simulink model "Simulink_Blocks"  (R2025b)
settings: Solver=FixedStepAuto  StartTime=0.0  StopTime=inf  RelTol=1e-3
undefined symbols (not defined in the file): Hermitian, j, jsin, magnitude, Skew, Symmetric
libraries: simulink x38, matrix_library x7
settings Model: SimulationMode=external  Creator=kueh_js  LastModifiedBy=kueh_js
settings OptimizationCC: OptimizeBlockIOStorage=off  EnhancedBackFolding=on  PassReuseOutputArgsThreshold=0.0  ZeroExternalMemoryAtStartup=off  ZeroInternalMemoryAtStartup=off  OptimizeBlockOrder=speed  DifferentSizesBufferReuse=on
settings DebuggingCC: ParameterTunabilityLossMsg=error
settings HardwareCC: ProdBitPerLong=64.0  ProdHWDeviceType=Intel->x86-64 (Linux 64)
settings SFSimCC: MATLABDynamicMemAlloc=off  SimTargetLang=C++  SimDLTargetLibrary=mkl-dnn
settings RTWCC: GenCodeOnly=on  Toolchain=GNU gcc/g++ | gmake (64-bit Linux)  TargetLang=C++
settings CodeAppCC: ForceParamTrailComments=on  OperatorAnnotations=on  MATLABSourceComments=on
settings GRTTargetCC: TargetLangStandard=C++20 (ISO)  MatFileLogging=off  CodeInterfacePackaging=C++ class

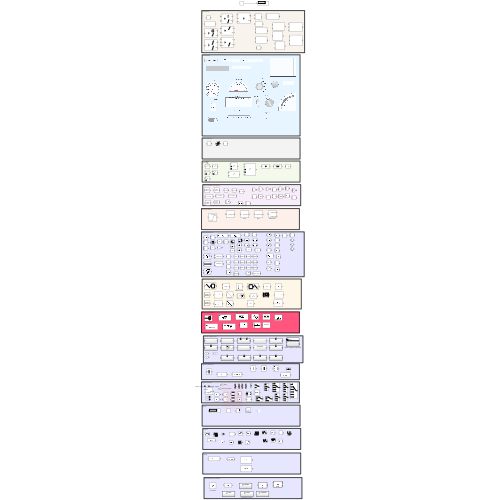
[thumbnail: Simulink's stored preview of the top-level diagram]
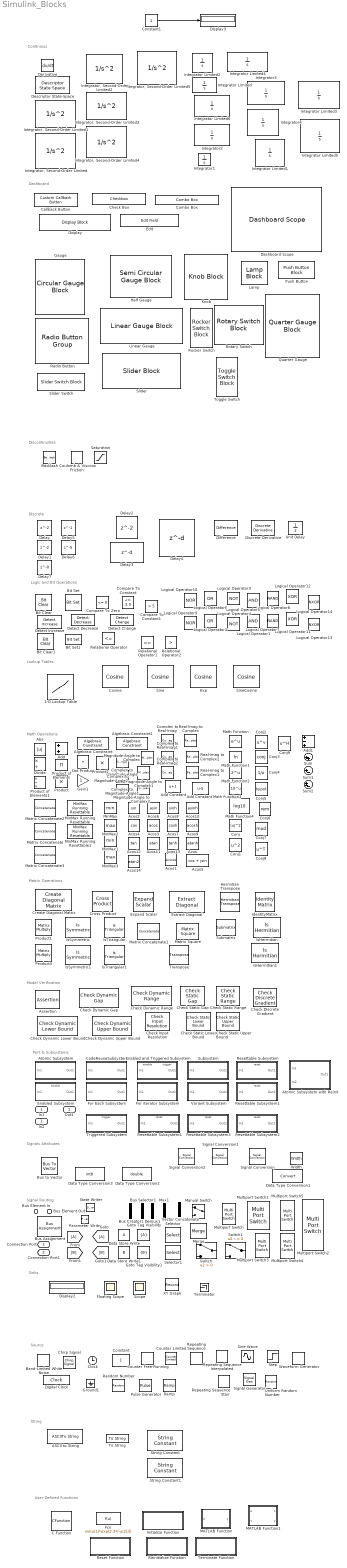
== system Simulink_Blocks ==
  note: Discontinuities
  note: Dashboard
  note: Continious
  note: Discrete
  note: Logic and Bit Operations
  note: Lookup Tables
  note: Math Operations
  note: Matrix Operations
  note: Model Verification
  note: Port & Subsystems
  note: Signals Attributes
  note: Signal Routing
  note: Sinks
  note: Source
  note: String
  note: User-Defined Functions
  In1 : Inport
  Bus Element In : Inport  Port=2  PortName=InBus  Element=signal1
  1-D Lookup Table : Lookup_n-D  NumberOfTableDimensions=1  BreakpointsForDimension1=[-5:5]  Table=tanh([-5:5])  InternalRulePriority=Speed  RndMeth=Simplest
  ASCII to String : ASCIIToString
  Abs : Abs  SaturateOnIntegerOverflow=off
  Acos : Trigonometry  Operator=atanh
  Acos1 : Trigonometry  Operator=sincos
  Acos10 : Trigonometry  Operator=asinh
  Acos11 : Trigonometry  Operator=atan
  Acos12 : Trigonometry  Operator=tan
  Acos13 : Trigonometry  Operator=tanh
  Acos14 : Trigonometry  Operator=atan2
  Acos2 : Trigonometry
  Acos3 : Trigonometry  Operator=acos
  Acos4 : Trigonometry  Operator=cos
  Acos5 : Trigonometry  Operator=cos + jsin
  Acos6 : Trigonometry  Operator=asin
  Acos7 : Trigonometry  Operator=cosh
  Acos8 : Trigonometry  Operator=sinh
  Acos9 : Trigonometry  Operator=acosh
  Add : Sum
  Add Constant : Bias  Bias=1  SaturateOnIntegerOverflow=off
  Add Constant1 : Bias  Bias=-5  SaturateOnIntegerOverflow=off
  Add1 : Sum  Inputs=+-+
  Algebraic Constraint : AlgebraicConstraint
  Algebraic Constraint1 : AlgebraicConstraint  Constraint=f(z) = z
  Assertion : Assertion
  Atomic Subsystem : Subsystem  TreatAsAtomicUnit=on
  Atomic Subsystem with Reinit : Subsystem  TreatAsAtomicUnit=on  ShowSubsystemReinitializePorts=on
  Backlash : Backlash
  Band-Limited White Noise : simulink/Sources/Band-Limited White Noise  Cov=[0.1]  Ts=0.1  seed=[23341]
  Bit Clear : simulink/Logic and Bit Operations/Bit Clear  iBit=0
  Bit Clear1 : simulink/Logic and Bit Operations/Bit Clear  iBit=3
  Bit Set : simulink/Logic and Bit Operations/Bit Set  iBit=0
  Bit Set1 : simulink/Logic and Bit Operations/Bit Set  iBit=2
  Bus Assignment : BusAssignment  AssignedSignals=signal1
  Bus Creator1 : BusCreator  Inputs=2
  Bus Selector1 : BusSelector  OutputSignals=signal1,signal2
  Bus to Vector : BusToVector
  C Function : CFunction
  Callback Button : CustomCallbackButton  Configuration="{\"components\":[{\"name\":\"BackgroundImageComponent\",\"settings\":{\"image\":{\"size\":[0,0],\"src\":\"default\",\"srcOrientation\":\"Right\"},\"position\":[0,0,1,1]}},{\"name\":\"ButtonStateComponent\",\"settings\":{\"buttonType\":\"momentary\",\"clickFcn\":\"\",\"onValue\":1,\"position\":[0,0,1,1],\"pressDelay\":\"500\",\"pressFcn\":\"\",\"repeatInterval\":\"0\",\"states\":[{\"horizontalAlignment\":\"center\",\"image\":{\"position\":[0,0,1,1],\"src\":\"default\",\"srcOrientation\":\"Right\"},\"label\":{\"color\":[0.01176470588,0.01176470588,0.01176470588,1],\"icon\":{\"size\":[0,0],\"src\":\"default\",\"srcOrientation\":\"Right\"},\"iconPlacement\":\"left\",\"text\":{\"content\":\"Callback Button\"}},\"labelOffset\":[0,0],\"verticalAlignment\":\"middle\"},{\"horizontalAlignment\":\"center\",\"image\":{\"position\":[0,0,1,1],\"src\":\"default\",\"srcOrientation\":\"Right\"},\"label\":{\"color\":[0.01176470588,0.01176470588,0.01176470588,1],\"icon\":{\"size\":[0,0],\"src\":\"default\",\"srcOrientation\":\"Right\"},\"iconPlacement\":\"left\",\"text\":{\"content\":\"Callback Button\"}},\"labelOffset\":[0,0],\"verticalAlignment\":\"middle\"},{\"horizontalAlignment\":\"center\",\"image\":{\"position\":[0,0,1,1],\"src\":\"default\",\"srcOrientation\":\"Right\"},\"label\":{\"color\":[0.01176470588,0.01176470588,0.01176470588,1],\"icon\":{\"size\":[0,0],\"src\":\"default\",\"srcOrientation\":\"Right\"},\"iconPlacement\":\"left\",\"text\":{\"content\":\"Callback Button\"}},\"labelOffset\":[0,0],\"verticalAlignment\":\"middle\"},{\"horizontalAlignment\":\"center\",\"image\":{\"position\":[0,0,1,1],\"src\":\"default\",\"srcOrientation\":\"Right\"},\"label\":{\"color\":[0.01176470588,0.01176470588,0.01176470588,1],\"icon\":{\"size\":[0,0],\"src\":\"default\",\"srcOrientation\":\"Right\"},\"iconPlacement\":\"left\",\"text\":{\"content\":\"Callback Button\"}},\"labelOffset\":[0,0],\"verticalAlignment\":\"middle\"}]}},{\"name\":\"ForegroundImageComponent\",\"settings\":{\"image\":{\"size\":[0,0],\"src\":\"default\",\"srcOrientation\":\"Right\"},\"isForeground\":1,\"position\":[0,0,1,1]}}],\"derived\":{\"blockParameters\":{\"AutoActivate\":true,\"ButtonText\":\"Callback Button\",\"ButtonType\":\"Momentary\",\"ClickFcn\":\"\",\"OnValue\":1,\"PressDelay\":\"500\",\"PressFcn\":\"\",\"RepeatInterval\":\"0\",\"fixedAspectRatio\":\"off\"}},\"settings\":{\"BindingType\":\"standalone\",\"autoActivate\":true,\"backgroundColor\":[244,244,244,1],\"backgroundOffset\":0.2,\"backgroundOpacity\":1,\"fixedAspectRatio\":\"off\",\"foregroundColor\":[0.01176470588,0.01176470588,0.01176470588,1],\"migratedFromLegacy\":true,\"useBackgroundColor\":true,\"variant\":\"callback\",\"version\":\"R2025a\"},\"type\":\"Button\"}"  CustomBackgroundColor="{\"color\":[0.9568627451,0.9568627451,0.9568627451],\"show\":true}"
  Check Discrete Gradient : simulink/Model Verification/Check Discrete Gradient  Description=| du / dt | < 1  gradient=1  enabled=on  stopWhenAssertionFail=on  export=off  icon=graphic
  Check Dynamic Gap : simulink/Model Verification/Check  Dynamic Gap  Description=u < min || max < u  enabled=on  stopWhenAssertionFail=on  export=off  icon=graphic
  Check Dynamic Range : simulink/Model Verification/Check  Dynamic Range  Description=min < u < max  enabled=on  stopWhenAssertionFail=on  export=off  icon=graphic
  Check Static Gap : simulink/Model Verification/Check  Static Gap  Description=u <= 0 || 100 <= u  max=100  max_included=on  min=0  min_included=on  enabled=on  stopWhenAssertionFail=on  export=off  icon=graphic
  Check Static Range : simulink/Model Verification/Check  Static Range  Description=0 <= u <= 100  max=100  max_included=on  min=0  min_included=on  enabled=on  stopWhenAssertionFail=on  export=off  icon=graphic
  Check Box : Checkbox  LabelPosition=Hide  ShowInitialText=on  Values=[0.0, 1.0]
  Check Dynamic Lower Bound : simulink/Model Verification/Check Dynamic  Lower Bound  Description=min < u  Enabled=on  stopWhenAssertionFail=on  export=off  icon=graphic
  Check Dynamic Upper Bound : simulink/Model Verification/Check Dynamic  Upper Bound  Description=u < max  enabled=on  stopWhenAssertionFail=on  export=off  icon=graphic
  Check Input Resolution : simulink/Model Verification/Check Input  Resolution  Description=-Inf < u < +Inf  resolution=1  enabled=on  stopWhenAssertionFail=on  export=off
  Check Static Lower Bound : simulink/Model Verification/Check Static  Lower Bound  Description=0 <= u  min=0  min_included=on  enabled=on  stopWhenAssertionFail=on  export=off  icon=graphic
  Check Static Upper Bound : simulink/Model Verification/Check Static  Upper Bound  Description=u <= 0  max=0  max_included=on  enabled=on  stopWhenAssertionFail=on  export=off  icon=graphic
  Chirp Signal : simulink/Sources/Chirp Signal  f1=0.1  T=100  f2=1
  Clock : Clock
  CodeReuseSubsystem : Subsystem  TreatAsAtomicUnit=on
      settings: RTWFcnNameOpts=Use subsystem name  RTWFileNameOpts=Use function name
  Combo Box : ComboBox  LabelPosition=Hide  SelectedLabel=Label2
  Compare To Constant : simulink/Logic and Bit Operations/Compare To Constant  relop=<=  const=3.0  OutDataTypeStr=boolean
  Compare To Constant1 : simulink/Logic and Bit Operations/Compare To Constant  relop=>  const=5  OutDataTypeStr=boolean
  Compare To Zero : simulink/Logic and Bit Operations/Compare To Zero  relop=<=  OutDataTypeStr=boolean
  Complex to Magnitude-Angle : ComplexToMagnitudeAngle
  Complex to Magnitude-Angle1 : ComplexToMagnitudeAngle  Output=Angle
  Complex to Magnitude-Angle2 : ComplexToMagnitudeAngle  Output=Magnitude
  Complex to Real-Imag : ComplexToRealImag
  Complex to Real-Imag1 : ComplexToRealImag  Output=Real
  Complex to Real-Imag2 : ComplexToRealImag  Output=Imag
  Conj : Math  Operator=magnitude^2
  Conj1 : Math  Operator=square
  Conj2 : Math  Operator=pow
  Conj3 : Math  Operator=conj
  Conj4 : Math  Operator=reciprocal
  Conj5 : Math  Operator=hypot
  Conj6 : Math  Operator=rem
  Conj7 : Math  Operator=mod
  Conj8 : Math  Operator=transpose
  Conj9 : Math  Operator=hermitian
  Constant : Constant
  Constant1 : Constant
  Cosine : simulink/Lookup Tables/Cosine  Formula=cos(2*pi*u)  NumDataPoints=(2^5)+1  OutputWordLength=16  InternalRulePriority=Speed
  Coulomb & Viscous Friction : simulink/Discontinuities/Coulomb & Viscous Friction  offset=[1 3 2 0]  gain=1
  Counter Free-Running : simulink/Sources/Counter Free-Running  NumBits=16  tsamp=-1
  Counter Limited : simulink/Sources/Counter Limited  uplimit=7  tsamp=-1
  Create Diagonal Matrix : matrix_library/Create Diagonal Matrix
      settings: LibrarySourceBlock=|
      | simulink/Matrix
      | Operations/Create Diagonal
      | Matrix
  Cross Product : matrix_library/Cross Product
  Dashboard Scope : DashboardScope  FontColor=[0.0, 0.0, 0.0]
  Data Store Write : DataStoreWrite  IndexOptions=Index vector (dialog)  Indices=1  OutputSizes=1
  Data Store Write1 : DataStoreWrite  DataStoreName=B  IndexOptions=Index vector (dialog)  Indices=1  OutputSizes=1
  Data Type Conversion1 : DataTypeConversion  SaturateOnIntegerOverflow=off  RndMeth=Floor
  Data Type Conversion2 : DataTypeConversion  OutDataTypeStr=double  SaturateOnIntegerOverflow=off  RndMeth=Floor
  Data Type Conversion3 : DataTypeConversion  OutDataTypeStr=int8  SaturateOnIntegerOverflow=off  RndMeth=Floor
  Delay : Delay
  Delay1 : Delay  ShowEnablePort=on
      settings: InputPortMap=u0,e6
  Delay2 : Delay  ExternalReset=Rising  ShowEnablePort=on
      settings: InputPortMap=u0,e6,r5
  Delay3 : Delay  DelayLengthSource=Input port
      settings: InputPortMap=u0,p1
  Delay4 : Delay  DelayLengthSource=Input port  InitialConditionSource=Input port  ExternalReset=Falling  ShowEnablePort=on
      settings: InputPortMap=u0,p1,e6,r5,p4
  Delay5 : Delay  DelayLength=1
  Delay6 : Delay  DelayLength=5  ShowEnablePort=on
      settings: InputPortMap=u0,e6
  Delay7 : Delay  DelayLength=0  ShowEnablePort=on
      settings: InputPortMap=u0,e6
  Demux1 : Demux  Outputs=2
  Derivative : Derivative
  Descriptor State-Space : DescriptorStateSpace
  Detect Change : simulink/Logic and Bit Operations/Detect Change  vinit=0  OutDataTypeStr=boolean
  Detect Decrease : simulink/Logic and Bit Operations/Detect Decrease  vinit=0.0  OutDataTypeStr=boolean
  Detect Increase : simulink/Logic and Bit Operations/Detect Increase  vinit=0  OutDataTypeStr=boolean
  Difference : simulink/Discrete/Difference  ICPrevInput=0.0  OutMin=[]  OutMax=[]  OutDataType=fixdt(1, 16)  OutScaling=2^-10  DoSatur=off
  Digital Clock : DigitalClock
  Discrete Derivative : simulink/Discrete/Discrete Derivative  gainval=1  ICPrevScaledInput=0  OutMin=[]  OutMax=[]  OutDataType=fixdt(1, 16)  OutScaling=2^-10  DoSatur=off
  Display : DisplayBlock  LabelPosition=Hide  Transparency=1  GridColor=[0.502, 0.502, 0.502]
  Display2 : Display
  Display3 : Display
  Divide : Product  Inputs=*/
  Dot Product : DotProduct  OutDataTypeStr=Inherit: Inherit via internal rule
  Edit : EditField  LabelPosition=Hide  ShowInitialText=on  Alignment=Center
  Enabled Subsystem : Subsystem  TreatAsAtomicUnit=on
  Enabled and Triggered Subsystem : Subsystem  TreatAsAtomicUnit=on
  Exp : simulink/Lookup Tables/Cosine  Formula=exp(j*2*pi*u)  NumDataPoints=(2^5)+1  OutputWordLength=16  InternalRulePriority=Speed
  Expand Scalar : ExpandScalar  OutputDimensions=6
  Extract Diagonal : matrix_library/Extract Diagonal
      settings: LibrarySourceBlock=|
      | simulink/Matrix
      | Operations/Extract Diagonal
  Fcn : Fcn  Expr=sin(u(1)*exp(2.3*(-u(2))))
  Floating Scope : Scope
      settings: IsFloating=on  Floating=on
  For Each Subsystem : Subsystem  TreatAsAtomicUnit=on
  For Iterator Subsystem : Subsystem  TreatAsAtomicUnit=on
  From : From
  Gain1 : Gain
  Gauge : CircularGaugeBlock  FontColor=[0.0, 0.0, 0.0]
  Goto : Goto
  Goto Tag Visibility : GotoTagVisibility
  Goto Tag Visibility1 : GotoTagVisibility  GotoTag=B
  Ground1 : Ground
  Half Gauge : SemiCircularGaugeBlock  FontColor=[0.0, 0.0, 0.0]
  Hermitian Transpose : matrix_library/Hermitian Transpose
      settings: LibrarySourceBlock=|
      | simulink/Matrix
      | Operations/Hermitian Transpose
  IdentityMatrix : IdentityMatrix
  In2 : InportShadow
  Initialize Function : Subsystem  TreatAsAtomicUnit=on
  Integrator Limited : Integrator  LimitOutput=on  UpperSaturationLimit=1  LowerSaturationLimit=0
  Integrator Limited1 : Integrator  ExternalReset=level hold  LimitOutput=on  UpperSaturationLimit=1  LowerSaturationLimit=0
  Integrator Limited2 : Integrator  InitialConditionSource=external  LimitOutput=on  UpperSaturationLimit=1  LowerSaturationLimit=0
  Integrator Limited3 : Integrator  ExternalReset=level  InitialConditionSource=external  UpperSaturationLimit=1  LowerSaturationLimit=0
  Integrator Limited4 : Integrator  ExternalReset=rising  InitialConditionSource=external  LimitOutput=on  UpperSaturationLimit=1  LowerSaturationLimit=0
  Integrator Limited5 : Integrator  ExternalReset=either  InitialConditionSource=external  UpperSaturationLimit=1  LowerSaturationLimit=0
  Integrator Limited6 : Integrator  ExternalReset=falling  LimitOutput=on  UpperSaturationLimit=1  LowerSaturationLimit=0
  "Integrator, Second-Order Limited" : SecondOrderIntegrator  LimitX=on  UpperLimitX=1  LowerLimitX=0  LimitDXDT=on
  "Integrator, Second-Order Limited1" : SecondOrderIntegrator  UpperLimitX=1  LowerLimitX=0  WrapX=on  LimitDXDT=on
  "Integrator, Second-Order Limited2" : SecondOrderIntegrator  ICSourceX=external  UpperLimitX=1  LowerLimitX=0  WrapX=on  LimitDXDT=on
  "Integrator, Second-Order Limited3" : SecondOrderIntegrator  ICSourceX=external  LimitX=on  UpperLimitX=1  LowerLimitX=0
  "Integrator, Second-Order Limited4" : SecondOrderIntegrator  ICSourceX=external  UpperLimitX=1  LowerLimitX=0  ICSourceDXDT=external  LimitDXDT=on
  "Integrator, Second-Order Limited5" : SecondOrderIntegrator  ICSourceX=external  UpperLimitX=1  LowerLimitX=0  ICSourceDXDT=external
  Integrator1 : Integrator
  Integrator2 : Integrator  InitialConditionSource=external
  Integrator3 : Integrator  InitialConditionSource=external  WrapState=on
  Integrator4 : Integrator  WrapState=on
  IsHermitian : IsHermitian
  IsHermitian1 : IsHermitian  Mode=Skew-Hermitian
  IsSymmetric : IsSymmetric
  IsSymmetric1 : IsSymmetric  Mode=Skew-Symmetric
  IsTriangular : IsTriangular
  IsTriangular1 : IsTriangular  Mode=Lower
  Knob : KnobBlock
  Lamp : LampBlock  LabelPosition=Hide  DefaultColor=[192.0, 192.0, 192.0]
  Linear Gauge : LinearGaugeBlock  FontColor=[0.0, 0.0, 0.0]
  Logical Operator1 : Logic  AllPortsSameDT=off  OutDataTypeStr=boolean
  Logical Operator10 : Logic  Operator=NOR  IconShape=distinctive  AllPortsSameDT=off  OutDataTypeStr=boolean
  Logical Operator11 : Logic  Operator=XOR  AllPortsSameDT=off  OutDataTypeStr=boolean
  Logical Operator12 : Logic  Operator=XOR  IconShape=distinctive  AllPortsSameDT=off  OutDataTypeStr=boolean
  Logical Operator13 : Logic  Operator=NXOR  AllPortsSameDT=off  OutDataTypeStr=boolean
  Logical Operator14 : Logic  Operator=NXOR  IconShape=distinctive  AllPortsSameDT=off  OutDataTypeStr=boolean
  Logical Operator2 : Logic  Operator=OR  AllPortsSameDT=off  OutDataTypeStr=boolean
  Logical Operator3 : Logic  Operator=NOT  IconShape=distinctive  AllPortsSameDT=off  OutDataTypeStr=boolean
  Logical Operator4 : Logic  Operator=NOT  AllPortsSameDT=off  OutDataTypeStr=boolean
  Logical Operator5 : Logic  IconShape=distinctive  AllPortsSameDT=off  OutDataTypeStr=boolean
  Logical Operator6 : Logic  Operator=OR  IconShape=distinctive  AllPortsSameDT=off  OutDataTypeStr=boolean
  Logical Operator7 : Logic  Operator=NAND  AllPortsSameDT=off  OutDataTypeStr=boolean
  Logical Operator8 : Logic  Operator=NAND  IconShape=distinctive  AllPortsSameDT=off  OutDataTypeStr=boolean
  Logical Operator9 : Logic  Operator=NOR  AllPortsSameDT=off  OutDataTypeStr=boolean
  MATLAB Function : MATLAB Function  TreatAsAtomicUnit=on
  MATLAB Function1 : MATLAB Function  TreatAsAtomicUnit=on
  Magnitude-Angle to Complex : MagnitudeAngleToComplex
  Magnitude-Angle to Complex1 : MagnitudeAngleToComplex  Input=Magnitude
  Magnitude-Angle to Complex2 : MagnitudeAngleToComplex  Input=Angle
  Manual Switch : ManualSwitch
  Math Function : Math
  Math Function1 : Math  Operator=log
  Math Function2 : Math  Operator=2^u
  Math Function3 : Math  Operator=10^u
  Math Function4 : Math  Operator=log10
  Matrix Concatenate : Concatenate  ConcatenateDimension=2
  Matrix Concatenate1 : Concatenate  Mode=Multidimensional array  ConcatenateDimension=2
  Matrix Concatenate2 : Concatenate  Mode=Multidimensional array  ConcatenateDimension=2
  Matrix Concatenate3 : Concatenate  Mode=Multidimensional array  ConcatenateDimension=3
  Matrix Square : matrix_library/Matrix Square  OutMin=[]  OutMax=[]
      settings: LibrarySourceBlock=|
      | simulink/Matrix
      | Operations/Matrix
      | Square
  Merge : Merge
  MinMax : MinMax
  MinMax Running Resettable : simulink/Math Operations/MinMax Running Resettable  Function=min  vinit=0.0
  MinMax Running Resettable1 : simulink/Math Operations/MinMax Running Resettable  Function=max  vinit=0.0
  MinMax1 : MinMax  Inputs=2
  MinMax2 : MinMax  Function=max
  MinMax3 : MinMax  Function=max  Inputs=3
  Multiport Switch : MultiPortSwitch  SaturateOnIntegerOverflow=off  InputSameDT=off
  Multiport Switch1 : MultiPortSwitch  Inputs=4  SaturateOnIntegerOverflow=off  InputSameDT=off
  Multiport Switch2 : MultiPortSwitch  Inputs=4  DataPortForDefault=Additional data port  SaturateOnIntegerOverflow=off  InputSameDT=off
  Multiport Switch3 : MultiPortSwitch  DataPortOrder=Zero-based contiguous  zeroidx=on  SaturateOnIntegerOverflow=off  InputSameDT=off
  Multiport Switch4 : MultiPortSwitch  DataPortOrder=Specify indices  DataPortIndices={6,8,15}  SaturateOnIntegerOverflow=off  InputSameDT=off
  Multiport Switch5 : MultiPortSwitch  DataPortOrder=Specify indices  DataPortIndices={6,8,15}  DataPortForDefault=Additional data port  SaturateOnIntegerOverflow=off  InputSameDT=off
  Mux1 : Mux  Inputs=2
  Parameter Writer : ParameterWriter  ParameterOwnerBlock=../Add Constant  ParameterName=Bias  ParameterInternalName=Bias
  Product : Product
  Product of Elements : Product  Inputs=*
  Product of Elements1 : Product  Inputs=*/*
  Product1 : Product  Multiplication=Matrix(*)
  Product2 : Product  Inputs=3
  Product3 : Product  Inputs=3  Multiplication=Matrix(*)
  Pulse Generator : DiscretePulseGenerator  PulseType=Time based  Period=10  PulseWidth=5
  Push Button : PushButtonBlock  IconOnColor=[0.0, 0.39215686274509803, 0.0]  IconOffColor=[0.0, 1.0, 0.0]
  Quarter Gauge : QuarterGaugeBlock  FontColor=[0.0, 0.0, 0.0]
  Radio Button : RadioButtonGroup  SelectedLabel=Label2  ButtonGroupName=Group
  Ramp : simulink/Sources/Ramp  slope=1  start=0  InitialOutput=0
  Random Number : RandomNumber  SampleTime=0.1
  Real-Imag to Complex : RealImagToComplex
  Real-Imag to Complex1 : RealImagToComplex  Input=Imag
  Real-Imag to Complex2 : RealImagToComplex  Input=Real
  Reinitialize Function : Subsystem  TreatAsAtomicUnit=on
  Relational Operator : RelationalOperator  Operator=<=  OutDataTypeStr=boolean  RndMeth=Simplest  InputSameDT=off
  Relational Operator1 : RelationalOperator  Operator===  OutDataTypeStr=boolean  RndMeth=Simplest  InputSameDT=off
  Relational Operator2 : RelationalOperator  Operator=>  OutDataTypeStr=boolean  RndMeth=Simplest  InputSameDT=off
  Repeating Sequence : simulink/Sources/Repeating Sequence  rep_seq_t=[0 2]  rep_seq_y=[0 2]
  Repeating Sequence Interpolated : simulink/Sources/Repeating Sequence Interpolated  OutValues=[3 1 4 2 1].'  TimeValues=[0 0.1 0.5 0.6 1].'  LookUpMeth=Interpolation-Use End Values  tsamp=0.01  OutMin=[]  OutMax=[]  OutDataTypeStr=double  OutputDataTypeScalingMode=double  OutDataType=fixdt(0,8)  OutScaling=2^-10
  Repeating Sequence Stair : simulink/Sources/Repeating Sequence Stair  OutValues=[3 1 4 2 1].'  tsamp=-1  OutMin=[]  OutMax=[]  OutDataTypeStr=double  OutputDataTypeScalingMode=double  OutDataType=fixdt(0,8)  ConRadixGroup=Best Precision: Vector-wise  OutScaling=2^-12
  Reset Function : Subsystem  TreatAsAtomicUnit=on
  Resettable Subsystem : Subsystem  TreatAsAtomicUnit=on
  Resettable Subsystem1 : Subsystem  TreatAsAtomicUnit=on
  Resettable Subsystem2 : Subsystem  TreatAsAtomicUnit=on
  Resettable Subsystem3 : Subsystem  TreatAsAtomicUnit=on
  Resettable Subsystem4 : Subsystem  TreatAsAtomicUnit=on
  Rocker Switch : RockerSwitchBlock
  Rotary Switch : RotarySwitchBlock
  Saturation : Saturate
  Scope : Scope
  Selector : Selector  InputPortWidth=3  IndexOptions=Index vector (dialog)  Indices=[1 3]  OutputSizes=1
  Selector1 : Selector  NumberOfDimensions=2  InputPortWidth=3  IndexOptions=Index vector (dialog),Index vector (dialog)  Indices=[1 3],1  OutputSizes=1,1
  Signal Conversion : SignalConversion  OverrideOpt=off
  Signal Conversion1 : SignalConversion  ConversionOutput=Virtual bus  OverrideOpt=off
  Signal Conversion2 : SignalConversion  ConversionOutput=Nonvirtual bus  OverrideOpt=off
  Signal Generator : SignalGenerator  Units=rad/sec
  Sine : simulink/Lookup Tables/Cosine  Formula=sin(2*pi*u)  NumDataPoints=(2^5)+1  OutputWordLength=16  InternalRulePriority=Speed
  Sine Wave : Sin  SampleTime=0
  SineCosine : simulink/Lookup Tables/Cosine  Formula=sin(2*pi*u) and cos(2*pi*u)  NumDataPoints=(2^5)+1  OutputWordLength=16  InternalRulePriority=Speed
  Slider : SliderBlock
  Slider Switch : SliderSwitchBlock
  State Writer : StateWriter  StateOwnerBlock=../Delay
  Step : Step  SampleTime=0
  String Constant : StringConstant
  String Constant1 : StringConstant  String="\"Test\""
  Submatrix : matrix_library/Submatrix  RowSpan=All rows  RowStartMode=Last  RowStartIndex=1  RowEndMode=Last  RowEndIndex=1  ColSpan=Range of columns  ColStartMode=First  ColStartIndex=1  ColEndMode=Last  ColEndIndex=1
  Subsystem : Subsystem
  Sum : Sum  Inputs=|++
  Sum1 : Sum  Inputs=|+-
  Sum2 : Sum  Inputs=|+--
  Switch : Switch  Criteria=u2 > Threshold  SaturateOnIntegerOverflow=off  InputSameDT=off
  Switch1 : Switch  Criteria=u2 ~= 0  SaturateOnIntegerOverflow=off  InputSameDT=off
  Terminate Function : Subsystem  TreatAsAtomicUnit=on
  Terminator : Terminator
  To String : ToString
  Toggle Switch : ToggleSwitchBlock
  Transpose : matrix_library/Transpose
  Triggered Subsystem : Subsystem  TreatAsAtomicUnit=on
  Uniform Random Number : UniformRandomNumber  SampleTime=0.1
  Unit Delay : UnitDelay  SampleTime=-1  HasFrameUpgradeWarning=on
  Variant Subsystem : Subsystem  Variant=on
  Vector Concatenate : Concatenate
  Waveform Generator : simulink/Sources/Waveform Generator  OutMin=[]  OutMax=[]  OutDataTypeStr=double  SelectedSignal=1  BlockNames=MultiportSwitch_e3df3653d217406  SampleTime=0.1
  Width : Width
  XY Graph : Record  NumPorts=2.0  FileSettingsInternal="{\"entries\":[{\"content\":{\"excelSettings\":{\"content\":{},\"type\":\"Streamout.ExcelSettings\"},\"parquetSettings\":{\"content\":{},\"type\":\"Streamout.ParquetSettings\"}},\"type\":\"Streamout.FileSettingStorage\",\"uuid\":\"\"}],\"packageUris\":[\"http:\\/\\/schema.mathworks.com\\/mf0\\/streamout_blocks\\/R2020a\"],\"version\":\"1.0\"}"  FrameSettings=[0, 0]  Layout=[1 1]  SignalsInternal="{\"entries\":[{\"content\":{\"signals\":[{\"content\":{\"blockPath\":[],\"dimensions\":[1],\"domain\":\"\",\"lineColor\":\"#a2142f\",\"plots\":[ 1 ],\"port\":1,\"signalID\":1,\"signalName\":\"XY Graph:1\"},\"type\":\"RecordBlkView.Signal\",\"uuid\":\"\"},{\"content\":{\"blockPath\":[],\"dimensions\":[1],\"domain\":\"\",\"lineColor\":\"#139fff\",\"plots\":[ 1 ],\"port\":2,\"signalID\":2,\"signalName\":\"XY Graph:2\"},\"type\":\"RecordBlkView.Signal\",\"uuid\":\"\"}]},\"type\":\"RecordBlkView.InputSignals\",\"uuid\":\"\"}],\"packageUris\":[\"http:\\/\\/schema.mathworks.com\\/mf0\\/streamout_blocks\\/R2020a\"],\"version\":\"1.0\"}"  VisualizationBindings="{\"xyplotplugin\":{\"info\":[{\"series\":[{\"bindingParametersList\":[{\"parameter\":\"X-Axis\",\"signalID\":1,\"signalName\":\"XY Graph:1\"},{\"parameter\":\"Y-Axis\",\"signalID\":2,\"signalName\":\"XY Graph:2\"}],\"seriesID\":0}],\"subplotID\":1}]}}"  CompatibilityTag=XY
  Connection Port : PMIOPort  Side=Left
  Connection Port1 : PMIOPort  Port=2  Side=Left
  Out1 : Outport
  Bus Element Out : Outport  Port=2  PortName=OutBus  Element=signal1
  wires:
  Constant1/1 -> Display3/1

== system Simulink_Blocks/Atomic Subsystem ==
  In1 : Inport
  Out1 : Outport
  wires:
  In1/1 -> Out1/1

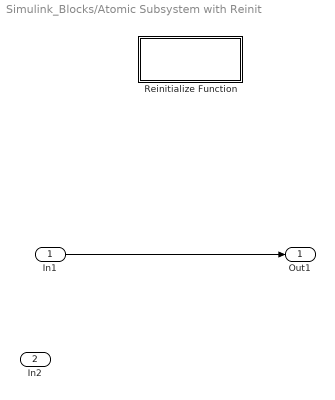
== system Simulink_Blocks/Atomic Subsystem with Reinit ==
  In1 : Inport
  In2 : Inport  Port=2
  Reinitialize Function : Subsystem  TreatAsAtomicUnit=on
  Out1 : Outport
  wires:
  In1/1 -> Out1/1

== system Simulink_Blocks/CodeReuseSubsystem ==
  In1 : Inport
  Out1 : Outport
  wires:
  In1/1 -> Out1/1

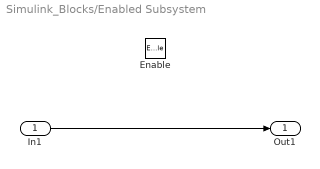
== system Simulink_Blocks/Enabled Subsystem ==
  In1 : Inport
  Enable : EnablePort
  Out1 : Outport
  wires:
  In1/1 -> Out1/1

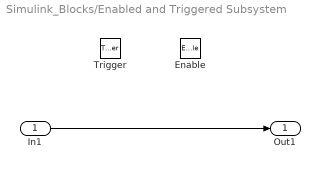
== system Simulink_Blocks/Enabled and Triggered Subsystem ==
  In1 : Inport
  Enable : EnablePort
  Trigger : TriggerPort  VariantControl=(inherit)
  Out1 : Outport
  wires:
  In1/1 -> Out1/1

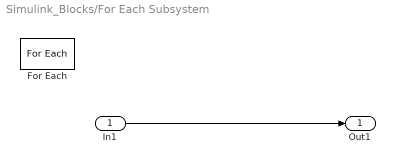
== system Simulink_Blocks/For Each Subsystem ==
  In1 : Inport  Partition=on  PartitionDimension=1  PartitionWidth=1  PartitionOffset=0
  For Each : ForEach  DisableCoverage=on
  Out1 : Outport  ConcatenationDimension=1
  wires:
  In1/1 -> Out1/1

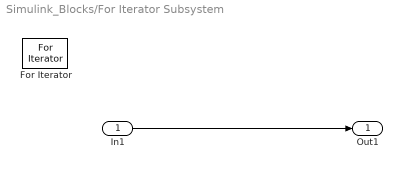
== system Simulink_Blocks/For Iterator Subsystem ==
  In1 : Inport
  For Iterator : ForIterator
  Out1 : Outport
  wires:
  In1/1 -> Out1/1

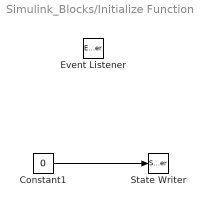
== system Simulink_Blocks/Initialize Function ==
  Constant1 : Constant  Value=0
  Event Listener : EventListener  DisableCoverage=on  EventName=reset
  State Writer : StateWriter
  wires:
  Constant1/1 -> State Writer/1

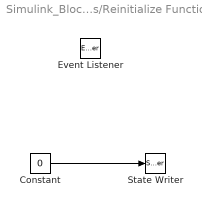
== system Simulink_Blocks/Reinitialize Function ==
  Constant : Constant  DisableCoverage=on  Value=0
  Event Listener : EventListener  DisableCoverage=on  EventType=Reinitialize  EventName=reinit
  State Writer : StateWriter  DisableCoverage=on
  wires:
  Constant/1 -> State Writer/1

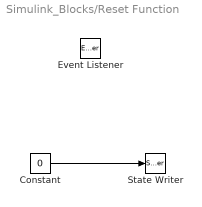
== system Simulink_Blocks/Reset Function ==
  Constant : Constant  Value=0
  Event Listener : EventListener  DisableCoverage=on  EventType=Reset  EventName=reset
  State Writer : StateWriter
  wires:
  Constant/1 -> State Writer/1

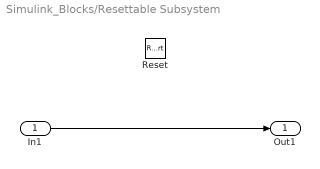
== system Simulink_Blocks/Resettable Subsystem ==
  In1 : Inport
  Reset : ResetPort  DisableCoverage=on
  Out1 : Outport
  wires:
  In1/1 -> Out1/1

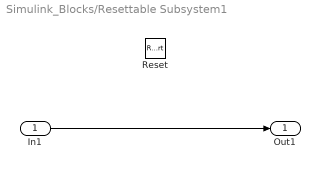
== system Simulink_Blocks/Resettable Subsystem1 ==
  In1 : Inport
  Reset : ResetPort  DisableCoverage=on  ResetTriggerType=falling
  Out1 : Outport
  wires:
  In1/1 -> Out1/1

== system Simulink_Blocks/Resettable Subsystem2 ==
  In1 : Inport
  Reset : ResetPort  DisableCoverage=on  ResetTriggerType=level hold
  Out1 : Outport
  wires:
  In1/1 -> Out1/1

== system Simulink_Blocks/Resettable Subsystem3 ==
  In1 : Inport
  Reset : ResetPort  DisableCoverage=on  ResetTriggerType=level
  Out1 : Outport
  wires:
  In1/1 -> Out1/1

== system Simulink_Blocks/Resettable Subsystem4 ==
  In1 : Inport
  Reset : ResetPort  DisableCoverage=on  ResetTriggerType=either
  Out1 : Outport
  wires:
  In1/1 -> Out1/1

== system Simulink_Blocks/Subsystem ==
  In1 : Inport
  Out1 : Outport
  wires:
  In1/1 -> Out1/1

== system Simulink_Blocks/Terminate Function ==
  Event Listener : EventListener  DisableCoverage=on  EventType=Terminate  EventName=reset
  State Reader : StateReader
  Terminator : Terminator
  wires:
  State Reader/1 -> Terminator/1

== system Simulink_Blocks/Triggered Subsystem ==
  In1 : Inport
  Trigger : TriggerPort  TriggerType=falling  VariantControl=(inherit)
  Out1 : Outport
  wires:
  In1/1 -> Out1/1

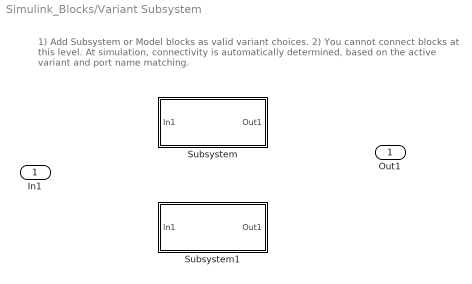
== system Simulink_Blocks/Variant Subsystem ==
  note: 1) Add Subsystem or Model blocks as valid variant choices.
      | 2) You cannot connect blocks at this level. At simulation, connectivity is automatically
      | determined, based on the active variant and port name matching.
  In1 : Inport
  Subsystem : Subsystem  VariantControl=true
  Subsystem1 : Subsystem  VariantControl=false
  Out1 : Outport

== system Simulink_Blocks/Atomic Subsystem with Reinit/Reinitialize Function ==
  Constant : Constant  DisableCoverage=on  Value=0
  Event Listener : EventListener  DisableCoverage=on  EventType=Reinitialize  EventName=reinit
  State Writer : StateWriter  DisableCoverage=on
  wires:
  Constant/1 -> State Writer/1

== system Simulink_Blocks/Variant Subsystem/Subsystem ==
  In1 : Inport
  Out1 : Outport

== system Simulink_Blocks/Variant Subsystem/Subsystem1 ==
  In1 : Inport
  Out1 : Outport

== matlab function Simulink_Blocks/MATLAB Function ==
  data: u input; y output
function y = fcn(u)

y = u;

== matlab function Simulink_Blocks/MATLAB Function1 ==
  data: x output; u input; y output; v input
function [x,y] = test(u,v)

y = u;
x=v;
